simulink model "beaver"  (Simulink 3.00)
settings: Solver=ode45  SolverMode=SingleTasking  StartTime=0.0  StopTime=60  MaxStep=10  RelTol=1e-8  AbsTol=1e-8
libraries: fdclib10 x1
settings Model: SaveTime=off  SaveOutput=off  RTWTemplateMakefile=grt_vc.tmf  LastModifiedBy=Dutchroll

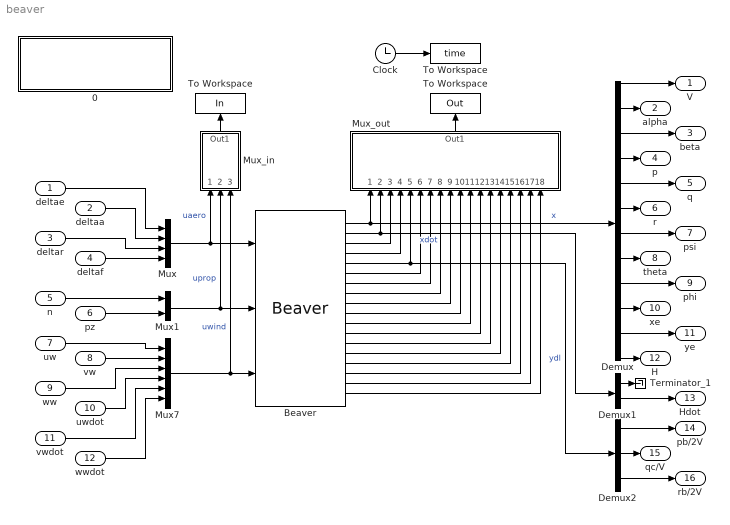
== system beaver ==
  deltae : Inport  Port=1  PortWidth=-1  SampleTime=-1  DataType=auto
      settings: SignalType=auto
  deltaa : Inport  Port=2  PortWidth=-1  SampleTime=-1  DataType=auto
      settings: SignalType=auto
  deltar : Inport  Port=3  PortWidth=-1  SampleTime=-1  DataType=auto
      settings: SignalType=auto
  deltaf : Inport  Port=4  PortWidth=-1  SampleTime=-1  DataType=auto
      settings: SignalType=auto
  n : Inport  Port=5  PortWidth=-1  SampleTime=-1  DataType=auto
      settings: SignalType=auto
  pz : Inport  Port=6  PortWidth=-1  SampleTime=-1  DataType=auto
      settings: SignalType=auto
  uw : Inport  Port=7  PortWidth=-1  SampleTime=-1  DataType=auto
      settings: SignalType=auto
  vw : Inport  Port=8  PortWidth=-1  SampleTime=-1  DataType=auto
      settings: SignalType=auto
  ww : Inport  Port=9  PortWidth=-1  SampleTime=-1  DataType=auto
      settings: SignalType=auto
  uwdot : Inport  Port=10  PortWidth=-1  SampleTime=-1  DataType=auto
      settings: SignalType=auto
  vwdot : Inport  Port=11  PortWidth=-1  SampleTime=-1  DataType=auto
      settings: SignalType=auto
  wwdot : Inport  Port=12  PortWidth=-1  SampleTime=-1  DataType=auto
      settings: SignalType=auto
  0 : Subsystem
      settings: OpenFcn=browse level1
      mask Display: disp('FDC Toolbox\nBEAVER, level 1\nM.O. Rauw, November 2004')
  Beaver : fdclib10/Beaver
  Clock : Clock
      settings: DisplayTime=off  Decimation=10
  Demux : Demux  Outputs=12
  Demux1 : Demux  Outputs=[11 1]
  Demux2 : Demux  Outputs=3
  Mux : Mux  Inputs=4
      settings: DisplayOption=none
  Mux1 : Mux  Inputs=2
      settings: DisplayOption=none
  Mux7 : Mux  Inputs=6
      settings: DisplayOption=none
  Mux_in : Subsystem  Orientation=up
      settings: OpenFcn=browse inputs
      mask Display: disp('Mux\nclick\n2x for\ninfo!')
  Mux_out : Subsystem  Orientation=up
      settings: OpenFcn=browse outputs
      mask Display: disp('Mux\n\nDouble-click for info!')
  Terminator_1 : Terminator
  To Workspace : ToWorkspace  VariableName=Out  SampleTime=0  SaveFormat=Matrix
      settings: Orientation=up  Buffer=5000
  "To Workspace " : ToWorkspace  VariableName=In  SampleTime=0  SaveFormat=Matrix
      settings: Orientation=up  Buffer=5000
  "To Workspace  " : ToWorkspace  VariableName=time  SampleTime=0  SaveFormat=Matrix
      settings: Buffer=5000
  V : Outport  Port=1
  alpha : Outport  Port=2
  beta : Outport  Port=3
  p : Outport  Port=4
  q : Outport  Port=5
  r : Outport  Port=6
  psi : Outport  Port=7
  theta : Outport  Port=8
  phi : Outport  Port=9
  xe : Outport  Port=10
  ye : Outport  Port=11
  H : Outport  Port=12
  Hdot : Outport  Port=13
  pb/2V : Outport  Port=14
  qc/V : Outport  Port=15
  rb/2V : Outport  Port=16
  wires:
  Mux_in/1(Out1) -> "To Workspace "/1
  Mux_out/1(Out1) -> To Workspace/1
  deltaf/1 -> Mux/4
  wwdot/1 -> Mux7/6
  uwdot/1 -> Mux7/4
  vw/1 -> Mux7/2
  pz/1 -> Mux1/2
  deltaa/1 -> Mux/2
  Demux1/1 -> Terminator_1/1
  Demux/1 -> V/1
  Demux/2 -> alpha/1
  Demux/3 -> beta/1
  Demux/4 -> p/1
  Demux/5 -> q/1
  Demux/6 -> r/1
  Demux/7 -> psi/1
  Demux/8 -> theta/1
  Demux/9 -> phi/1
  Demux/12 -> H/1
  Demux/11 -> ye/1
  Demux/10 -> xe/1
  Demux1/2 -> Hdot/1
  Demux2/1 -> pb/2V/1
  Demux2/2 -> qc/V/1
  Demux2/3 -> rb/2V/1
  Mux7/1 -> Beaver/3, Mux_in/3(In3)  "uwind"
  Mux1/1 -> Beaver/2, Mux_in/2(In2)  "uprop"
  Mux/1 -> Beaver/1, Mux_in/1(In1)  "uaero"
  Beaver/2 -> Mux_out/2(In2), Demux1/1  "xdot"
  Beaver/15 -> Mux_out/15(In15)
  Beaver/14 -> Mux_out/14(In14)
  Beaver/13 -> Mux_out/13(In13)
  Beaver/12 -> Mux_out/12(In12)
  Beaver/11 -> Mux_out/11(In11)
  Beaver/10 -> Mux_out/10(In10)
  Beaver/9 -> Mux_out/9(In9)
  Beaver/8 -> Mux_out/8(In8)
  Beaver/7 -> Mux_out/7(In7)
  Beaver/6 -> Mux_out/6(In6)
  Beaver/5 -> Demux2/1, Mux_out/5(In5)  "ydl"
  Beaver/16 -> Mux_out/16(In16)
  Beaver/3 -> Mux_out/3(In3)
  Beaver/1 -> Demux/1, Mux_out/1(In1)  "x"
  Beaver/4 -> Mux_out/4(In4)
  Beaver/17 -> Mux_out/17(In17)
  Beaver/18 -> Mux_out/18(In18)
  vwdot/1 -> Mux7/5
  ww/1 -> Mux7/3
  uw/1 -> Mux7/1
  n/1 -> Mux1/1
  deltae/1 -> Mux/1
  deltar/1 -> Mux/3
  Clock/1 -> "To Workspace  "/1

== system beaver/0 ==

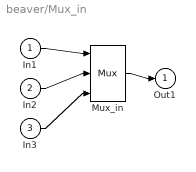
== system beaver/Mux_in ==
  In1 : Inport  Port=1  PortWidth=-1  SampleTime=-1  DataType=auto
      settings: SignalType=auto
  In2 : Inport  Port=2  PortWidth=-1  SampleTime=-1  DataType=auto
      settings: SignalType=auto
  In3 : Inport  Port=3  PortWidth=-1  SampleTime=-1  DataType=auto
      settings: SignalType=auto
  Mux_in : Mux  Inputs=[4 2 6]
      settings: DisplayOption=none
  Out1 : Outport  Port=1
  wires:
  In1/1 -> Mux_in/1
  In2/1 -> Mux_in/2
  In3/1 -> Mux_in/3
  Mux_in/1 -> Out1/1

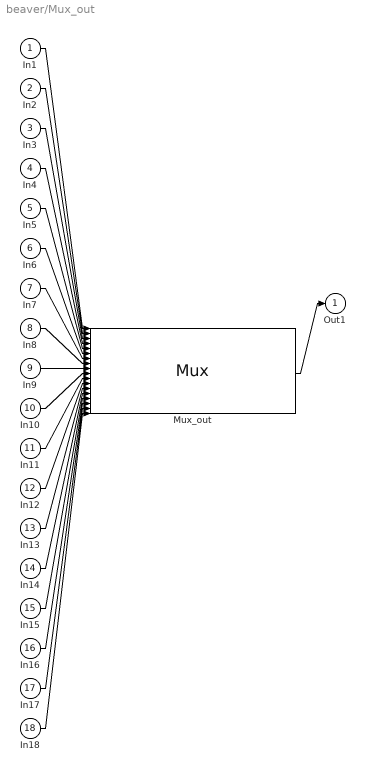
== system beaver/Mux_out ==
  In1 : Inport  Port=1  PortWidth=-1  SampleTime=-1  DataType=auto
      settings: SignalType=auto
  In2 : Inport  Port=2  PortWidth=-1  SampleTime=-1  DataType=auto
      settings: SignalType=auto
  In3 : Inport  Port=3  PortWidth=-1  SampleTime=-1  DataType=auto
      settings: SignalType=auto
  In4 : Inport  Port=4  PortWidth=-1  SampleTime=-1  DataType=auto
      settings: SignalType=auto
  In5 : Inport  Port=5  PortWidth=-1  SampleTime=-1  DataType=auto
      settings: SignalType=auto
  In6 : Inport  Port=6  PortWidth=-1  SampleTime=-1  DataType=auto
      settings: SignalType=auto
  In7 : Inport  Port=7  PortWidth=-1  SampleTime=-1  DataType=auto
      settings: SignalType=auto
  In8 : Inport  Port=8  PortWidth=-1  SampleTime=-1  DataType=auto
      settings: SignalType=auto
  In9 : Inport  Port=9  PortWidth=-1  SampleTime=-1  DataType=auto
      settings: SignalType=auto
  In10 : Inport  Port=10  PortWidth=-1  SampleTime=-1  DataType=auto
      settings: SignalType=auto
  In11 : Inport  Port=11  PortWidth=-1  SampleTime=-1  DataType=auto
      settings: SignalType=auto
  In12 : Inport  Port=12  PortWidth=-1  SampleTime=-1  DataType=auto
      settings: SignalType=auto
  In13 : Inport  Port=13  PortWidth=-1  SampleTime=-1  DataType=auto
      settings: SignalType=auto
  In14 : Inport  Port=14  PortWidth=-1  SampleTime=-1  DataType=auto
      settings: SignalType=auto
  In15 : Inport  Port=15  PortWidth=-1  SampleTime=-1  DataType=auto
      settings: SignalType=auto
  In16 : Inport  Port=16  PortWidth=-1  SampleTime=-1  DataType=auto
      settings: SignalType=auto
  In17 : Inport  Port=17  PortWidth=-1  SampleTime=-1  DataType=auto
      settings: SignalType=auto
  In18 : Inport  Port=18  PortWidth=-1  SampleTime=-1  DataType=auto
      settings: SignalType=auto
  Mux_out : Mux  Inputs=[12 12 3 3 3 4 2 6 6 6 6 6 3 3 5 3 3 3]
      settings: DisplayOption=none
  Out1 : Outport  Port=1
  wires:
  In1/1 -> Mux_out/1
  In2/1 -> Mux_out/2
  In3/1 -> Mux_out/3
  In4/1 -> Mux_out/4
  In5/1 -> Mux_out/5
  In6/1 -> Mux_out/6
  In7/1 -> Mux_out/7
  In8/1 -> Mux_out/8
  In9/1 -> Mux_out/9
  In10/1 -> Mux_out/10
  In11/1 -> Mux_out/11
  In12/1 -> Mux_out/12
  In13/1 -> Mux_out/13
  In14/1 -> Mux_out/14
  In15/1 -> Mux_out/15
  In16/1 -> Mux_out/16
  In17/1 -> Mux_out/17
  In18/1 -> Mux_out/18
  Mux_out/1 -> Out1/1
